simulink model "PMSM_FOC_Tractio"  (R2019b)
settings: Solver=FixedStepAuto  StartTime=0.0  StopTime=10  RelTol=1e-3
model workspace (MAT data in the model file):
  wc : Simulink.Parameter (value not decoded)
values from neighbouring files (symbols this model uses):
  CL_Param = tmp_CL_Param    [PMSM_Parameters.m]
  Cosine_table = [1,0.999995293095708,0.999990587122738,0.999985881149769,0.999981174245477,0.999967055395246,0.999952936545014,0.999938818626106,0.999924698844552,0.999901168979704,0.999877639114857,0.999854108318687,0.999830577522516,0.999797635711730,0.999764694832265,0.999731753021479,0.999698810279369,0.999656459316611,0.999614108353853,0.999571758322418,0.999529405497015,0.999477646313608,0.999425887130201,0 ...(+75635 chars)    [Motor_Table.m]
  ctrlParamsPI = tmp_ctrlParamsPI    [PMSM_Parameters.m]
  Flux_weak = tmp_Fluxweak_struct    [PMSM_Parameters.m]
  Hall_Parameter = tmp_Hall_struct    [PMSM_Parameters.m]
  HFI = tmp_HFI_struct    [PMSM_Parameters.m]
  inverter = struct    [PMSM_Parameters.m]
  MTPA_id_table = [-1.39452500000000,-1.36697494250000,-1.33970177000000,-1.31270548250000,-1.28598608000000,-1.25954356250000,-1.23337793000000,-1.20748918250000,-1.18187732000000,-1.15654234250000,-1.13148425000000,-1.10670304250000,-1.08219872000000,-1.05797128250000,-1.03402073000000,-1.01034706250000,-0.986950280000000,-0.963830382500000,-0.940987370000000,-0.918421242500000,-0.896132000000000,-0.8741196425000 ...(+3439 chars)    [Motor_Table.m]
  MTPA_iq_table = [-10.2740250000000,-10.1791705677750,-10.0840783722000,-9.98875081492500,-9.89319029760000,-9.79739922187500,-9.70137998940000,-9.60513500182500,-9.50866666080000,-9.41197736797500,-9.31506952500000,-9.21794553352500,-9.12060779520000,-9.02305871167500,-8.92530068460000,-8.82733611562500,-8.72916740640000,-8.63079695857500,-8.53222717380000,-8.43346045372500,-8.33449920000000,-8.23534581427500,-8. ...(+3121 chars)    [Motor_Table.m]
  MTPA_Te_Max = single(1.50)    [Motor_Table.m]
  MTPA_Te_Min = single(-1.50)    [Motor_Table.m]
  OPL_Param = tmp_OPL_Param    [PMSM_Parameters.m]
  pmsm = struct    [PMSM_Parameters.m]
  Resolver_Parameter = tmp_Resolver_struct    [PMSM_Parameters.m]
  Sine_table = [0,0.00153398793190718,0.00306797679513693,0.00460196565836668,0.00613595545291901,0.00766988657414913,0.00920381769537926,0.0107377488166094,0.0122716808691621,0.0138054965063930,0.0153393121436238,0.0168731296434999,0.0184069443494082,0.0199405867606401,0.0214742291718721,0.0230078706517816,0.0245415139943361,0.0260749254375696,0.0276083368808031,0.0291417483240366,0.0306751597672701,0.032208281 ...(+75648 chars)    [Motor_Table.m]
  SMO = temp_SMO    [PMSM_Parameters.m]
undefined symbols (not defined in the file or in its folder): DiscIntNeverNeededParam, Kiv, Kiw, Kpv, Kpw, magnitude, sigbuilder_block, SVPWM, Vdc
libraries: powerlib x29, fl_lib x18, simulink x10, nesl_utility x7, eeGeneralControl x4, dspstat3 x3, eeDiscretePi x2, powerlib_extras x1, ee_lib x1
(part 4 of 6)

== system PMSM_FOC_Tractio/Motor_Control/Motor_Control_Funtion/FOC_Control_100us/FOC/D_Current_PI ==
  Current_Command : Inport
  Current_Measured : Inport  Port=2
  Add2 : Sum  Inputs=|+-
  ID_Control : Subsystem
  Vd_voltage : Outport  VectorParamsAs1DForOutWhenUnconnected=off
  wires:
  Current_Command/1 -> Add2/1
  Current_Measured/1 -> Add2/2
  Add2/1 -> ID_Control/1(Err)  "currentControlError"
  ID_Control/1(PI_Out) -> Vd_voltage/1

== system PMSM_FOC_Tractio/Motor_Control/Motor_Control_Funtion/FOC_Control_100us/FOC/Flux_weakening  ==
  Enable : Inport
  Vd : Inport  Port=2
  Vq : Inport  Port=3
  Id : Inport  Port=4
  Iq : Inport  Port=5
  If1 : If  IfExpression=u1 ==1
  Merge : Merge
  Merge1 : Merge
  Subsystem : Subsystem
  Subsystem1 : Subsystem
  Id_ref : Outport
  Iq_ref : Outport  Port=2
  wires:
  Enable/1 -> If1/1
  If1/1 -> Subsystem/Action
  If1/2 -> Subsystem1/Action
  Id/1 -> Subsystem/3(Id), Subsystem1/1(Id)
  Iq/1 -> Subsystem/4(Iq), Subsystem1/2(Iq)
  Vd/1 -> Subsystem/1(Vd)
  Vq/1 -> Subsystem/2(Vq)
  Subsystem/1(Id_ref) -> Merge/1
  Subsystem1/1(Id_ref) -> Merge/2
  Subsystem/2(Iq_ref) -> Merge1/1
  Subsystem1/2(Iq_ref) -> Merge1/2
  Merge1/1 -> Iq_ref/1
  Merge/1 -> Id_ref/1

== system PMSM_FOC_Tractio/Motor_Control/Motor_Control_Funtion/FOC_Control_100us/FOC/HF_Observer ==
  Ialpha-beta : Inport
  Phase_CurrentABC : Inport  Port=2  PortDimensions=3
  Id : Inport  Port=3
  HFI_Enalble : Constant  Value=HFI.Func_Enable  OutDataTypeStr=uint8
  HFI_Function : Subsystem
      settings: RTWSystemCode=Nonreusable function  RTWFcnNameOpts=Use subsystem name
  If1 : If  IfExpression=u1==1  ShowElse=off
  RUN_State : Outport
  HFI_State : Outport  Port=2
  HFI_signal : Outport  Port=3
  speed_est : Outport  Port=4
  theta_est : Outport  Port=5
  Ualpha : Outport  Port=6
  Ubeta : Outport  Port=7
  IPD_Theta : Outport  Port=8
  wires:
  HFI_Function/1(RUN_State) -> RUN_State/1
  HFI_Function/3(HFI_signal) -> HFI_signal/1
  HFI_Function/4(speed_est) -> speed_est/1
  HFI_Function/5(theta_est) -> theta_est/1
  HFI_Function/7(Ubeta) -> Ubeta/1
  HFI_Function/6(Ualpha) -> Ualpha/1
  Id/1 -> HFI_Function/3(Id)
  Phase_CurrentABC/1 -> HFI_Function/2(Phase_CurrentABC)  "Phase_CurrentABC"
  Ialpha-beta/1 -> HFI_Function/1(Ialpha-beta)
  HFI_Enalble/1 -> If1/1
  If1/1 -> HFI_Function/Action
  HFI_Function/2(HFI_State) -> HFI_State/1
  HFI_Function/8(IPD_Theta) -> IPD_Theta/1

== system PMSM_FOC_Tractio/Motor_Control/Motor_Control_Funtion/FOC_Control_100us/FOC/Inverse_Park_Transform ==
  D : Inport
  Q : Inport  Port=2
  Sin_Coefficient : Inport  Port=3
  Cos_Coefficient : Inport  Port=4
  Add1 : Sum  Inputs=+-  OutDataTypeStr=Inherit: Same as first input
  Add2 : Sum  OutDataTypeStr=Inherit: Same as first input
  Cos_Coefficient1 : InportShadow  Port=4
  Product{1..4} (4 alike) : Product  RndMeth=Simplest  OutDataTypeStr=Inherit: Same as first input
  Sin_Coefficient1 : InportShadow  Port=3
  Alpha : Outport  VectorParamsAs1DForOutWhenUnconnected=off
  Beta : Outport  Port=2  VectorParamsAs1DForOutWhenUnconnected=off
  wires:
  Add2/1 -> Beta/1
  Add1/1 -> Alpha/1
  Product3/1 -> Add2/1
  Product4/1 -> Add2/2
  Product1/1 -> Add1/1
  Product2/1 -> Add1/2
  Cos_Coefficient1/1 -> Product4/2
  Sin_Coefficient/1 -> Product2/2
  D/1 -> Product3/1, Product1/1
  Q/1 -> Product2/1, Product4/1
  Sin_Coefficient1/1 -> Product3/2
  Cos_Coefficient/1 -> Product1/2

== system PMSM_FOC_Tractio/Motor_Control/Motor_Control_Funtion/FOC_Control_100us/FOC/Park_Transform ==
  Alpha : Inport
  Beta : Inport  Port=2
  Sin_Coefficient : Inport  Port=3
  Cos_Coefficient : Inport  Port=4
  Add1 : Sum  OutDataTypeStr=Inherit: Same as first input
  Add2 : Sum  Inputs=-+  OutDataTypeStr=Inherit: Same as first input
  Alpha1 : InportShadow
  Beta1 : InportShadow  Port=2
  Cos_Coefficient1 : InportShadow  Port=4
  Produc3t : Product  RndMeth=Simplest  OutDataTypeStr=Inherit: Same as first input
  Product1 : Product  RndMeth=Simplest  OutDataTypeStr=Inherit: Same as first input
  Product2 : Product  RndMeth=Simplest  OutDataTypeStr=Inherit: Same as first input
  Product4 : Product  RndMeth=Simplest  OutDataTypeStr=Inherit: Same as first input
  Sin_Coefficient1 : InportShadow  Port=3
  D : Outport  VectorParamsAs1DForOutWhenUnconnected=off
  Q : Outport  Port=2  VectorParamsAs1DForOutWhenUnconnected=off
  wires:
  Produc3t/1 -> Add2/1
  Product4/1 -> Add2/2
  Product1/1 -> Add1/1
  Product2/1 -> Add1/2
  Alpha1/1 -> Produc3t/1
  Sin_Coefficient1/1 -> Produc3t/2
  Cos_Coefficient1/1 -> Product4/2
  Beta1/1 -> Product4/1
  Alpha/1 -> Product1/1
  Cos_Coefficient/1 -> Product1/2
  Beta/1 -> Product2/1
  Sin_Coefficient/1 -> Product2/2
  Add1/1 -> D/1
  Add2/1 -> Q/1

== system PMSM_FOC_Tractio/Motor_Control/Motor_Control_Funtion/FOC_Control_100us/FOC/Q_Current_PI ==
  Current_Command : Inport
  Current_Measured : Inport  Port=2
  Add2 : Sum  Inputs=|+-
  IQ_Control : Subsystem
  Vq_voltage : Outport  VectorParamsAs1DForOutWhenUnconnected=off
  wires:
  Current_Command/1 -> Add2/1
  Current_Measured/1 -> Add2/2
  Add2/1 -> IQ_Control/1(Err)  "currentControlError"
  IQ_Control/1(PI_Out) -> Vq_voltage/1

== system PMSM_FOC_Tractio/Motor_Control/Motor_Control_Funtion/FOC_Control_100us/FOC/SVPWM ==
  Valpha : Inport
  Vbeta : Inport  Port=2
  Vdc : Inport  Port=3
  Ts : Inport  Port=4
  Gain : Gain  Gain=83990000
  Gain2 : Gain  Gain=83990000
  Gain3 : Gain  Gain=83990000
  N Sector  Caculate : Subsystem  TreatAsAtomicUnit=on
  T1 T2  Caculate : Subsystem  TreatAsAtomicUnit=on
  Tcm calculate : Subsystem  TreatAsAtomicUnit=on
  XYZ Caculate : Subsystem  TreatAsAtomicUnit=on
  Ta : Outport
  Tb : Outport  Port=2
  Tc : Outport  Port=3
  wires:
  Tcm calculate/2(Tcm2) -> Gain2/1
  Tcm calculate/3(Tcm3) -> Gain3/1
  Tcm calculate/1(Tcm1) -> Gain/1
  T1 T2  Caculate/2(T2) -> Tcm calculate/3(T2)
  XYZ Caculate/1(X) -> T1 T2  Caculate/2(X)
  N Sector  Caculate/1(N) -> T1 T2  Caculate/1(N), Tcm calculate/1(N)
  Vdc/1 -> XYZ Caculate/3(Udc)
  T1 T2  Caculate/1(T1) -> Tcm calculate/2(T1)
  XYZ Caculate/3(Z) -> T1 T2  Caculate/4(Z)
  XYZ Caculate/2(Y) -> T1 T2  Caculate/3(Y)
  Valpha/1 -> N Sector  Caculate/2(Ualf), XYZ Caculate/1(Ualfpa)
  Vbeta/1 -> N Sector  Caculate/1(Ubelta), XYZ Caculate/2(Ubelta)
  Ts/1 -> T1 T2  Caculate/5(Tpwm), Tcm calculate/4(Tpwm), XYZ Caculate/4(Tpwm)
  Gain/1 -> Ta/1
  Gain3/1 -> Tc/1
  Gain2/1 -> Tb/1

== system PMSM_FOC_Tractio/Motor_Control/Motor_Control_Funtion/FOC_Control_100us/FOC/Set_Idq ==
  HFI_state : Inport
  Id_Command : Inport  Port=2
  Iq_Command : Inport  Port=3
  Constant1 : Constant  Value=0  OutDataTypeStr=single
  Constant2 : Constant  Value=0  OutDataTypeStr=single
  If1 : If  IfExpression=u1==2 | u1==1
  Merge : Merge
  Merge1 : Merge
  Set_Idq : Subsystem  TreatAsAtomicUnit=on
      settings: RTWSystemCode=Nonreusable function  RTWFcnNameOpts=Use subsystem name
  Set_Idq1 : Subsystem  TreatAsAtomicUnit=on
      settings: RTWSystemCode=Nonreusable function  RTWFcnNameOpts=Use subsystem name
  Id : Outport  VectorParamsAs1DForOutWhenUnconnected=off
  Iq : Outport  Port=2  VectorParamsAs1DForOutWhenUnconnected=off
  wires:
  HFI_state/1 -> If1/1
  Constant2/1 -> Set_Idq/1(Id_Command)
  Constant1/1 -> Set_Idq/2(Iq_Command)
  Id_Command/1 -> Set_Idq1/1(Id_Command)
  Iq_Command/1 -> Set_Idq1/2(Iq_Command)
  If1/1 -> Set_Idq/Action
  If1/2 -> Set_Idq1/Action
  Set_Idq/1(Id) -> Merge/1
  Set_Idq1/1(Id) -> Merge/2
  Merge/1 -> Id/1
  Set_Idq/2(Iq) -> Merge1/1
  Set_Idq1/2(Iq) -> Merge1/2
  Merge1/1 -> Iq/1

== system PMSM_FOC_Tractio/Motor_Control/Motor_Control_Funtion/FOC_Control_100us/FOC/Sine_Cosine ==
  note: Sine Cosine Coefficients
  P : Inport
  Cosine : Lookup_n-D  NumberOfTableDimensions=1  LookupTableObject=''  BreakpointsForDimension1=[0:2*pi/4095:2*pi]  BreakpointsForDimension1FirstPoint=10  BreakpointsForDimension2FirstPoint=10  BreakpointsForDimension1Spacing=12  BreakpointsForDimension2Spacing=12  IndexSearchMethod=Evenly spaced points  Table=Cosine_table  InterpMethod=Flat  DiagnosticForOutOfRangeInput=Error  InternalRulePriority=Speed  RndMeth=Simplest  InputSameDT=on
  Saturation : Saturate  UpperLimit=2*pi-0.0001  LowerLimit=0+0.0001
  Scope : Scope  NumInputPorts=2
  Sine : Lookup_n-D  NumberOfTableDimensions=1  LookupTableObject=''  BreakpointsForDimension1=[0:2*pi/4095:2*pi]  BreakpointsForDimension1FirstPoint=10  BreakpointsForDimension2FirstPoint=10  BreakpointsForDimension1Spacing=12  BreakpointsForDimension2Spacing=12  IndexSearchMethod=Evenly spaced points  Table=Sine_table  InterpMethod=Flat  DiagnosticForOutOfRangeInput=Error  InternalRulePriority=Speed  RndMeth=Simplest  InputSameDT=on
  Sin : Outport  VectorParamsAs1DForOutWhenUnconnected=off
  Cos : Outport  Port=2  VectorParamsAs1DForOutWhenUnconnected=off
  wires:
  P/1 -> Saturation/1  "position"
  Sine/1 -> Scope/1, Sin/1
  Cosine/1 -> Scope/2, Cos/1
  Saturation/1 -> Cosine/1, Sine/1

== system PMSM_FOC_Tractio/Motor_Control/Motor_Control_Funtion/FOC_Control_100us/FOC/Subsystem1 ==
  HFI_State : Inport
  HFI_Ualpha : Inport  Port=2
  HFI_Ubeta : Inport  Port=3
  Ualpha : Inport  Port=4
  Ubeta : Inport  Port=5
  If Action Subsystem1 : Subsystem  TreatAsAtomicUnit=on
  If Action Subsystem2 : Subsystem  TreatAsAtomicUnit=on
  If1 : If  IfExpression=(u1<3)&(u1>0)
  Merge : Merge
  Merge1 : Merge
  Ualpha_out : Outport
  Ubeta_out : Outport  Port=2
  wires:
  If1/1 -> If Action Subsystem2/Action
  If1/2 -> If Action Subsystem1/Action
  HFI_Ualpha/1 -> If Action Subsystem2/1(In1)
  HFI_Ubeta/1 -> If Action Subsystem2/2(In2)
  Ualpha/1 -> If Action Subsystem1/1(In1)
  Ubeta/1 -> If Action Subsystem1/2(In2)
  If Action Subsystem2/1(Out1) -> Merge/1
  If Action Subsystem1/1(Out1) -> Merge/2
  If Action Subsystem2/2(Out2) -> Merge1/1
  If Action Subsystem1/2(Out2) -> Merge1/2
  Merge/1 -> Ualpha_out/1
  Merge1/1 -> Ubeta_out/1
  HFI_State/1 -> If1/1

== system PMSM_FOC_Tractio/Motor_Control/Motor_Control_Funtion/FOC_Control_100us/Iq_selector/Subsystem ==
  In1 : Inport
  Action Port : ActionPort  ActionPortLabel=if(u1 ==2 | u1 ==3)
  Out1 : Outport
  wires:
  In1/1 -> Out1/1

== system PMSM_FOC_Tractio/Motor_Control/Motor_Control_Funtion/FOC_Control_100us/Iq_selector/Subsystem1 ==
  In1 : Inport
  Action Port : ActionPort  ActionPortLabel=else
  Out1 : Outport
  wires:
  In1/1 -> Out1/1

== system PMSM_FOC_Tractio/PMSM/Control/Control/Commutation/Bit concatenate ==
  u : Inport
  Gain : Gain  Gain=[4 2 1]  Multiplication=Matrix(K*u)
  Sum of Elements : Sum  Inputs=+
  y : Outport  VectorParamsAs1DForOutWhenUnconnected=off
  wires:
  u/1 -> Gain/1
  Gain/1 -> Sum of Elements/1
  Sum of Elements/1 -> y/1

== system PMSM_FOC_Tractio/PMSM/SpeedAndAngle/ACC_OMG/Six_point/Sector_1 ==
  Action Port : ActionPort  ActionPortLabel=case [ 1 ]:
  Add : Sum
  Constant : Constant  Value=Hall_Parameter.Sector_1  OutDataTypeStr=single
  Constant1 : Constant  Value=Hall_Parameter.shift  OutDataTypeStr=single
  Angle_0 : Outport
  wires:
  Constant/1 -> Add/1
  Constant1/1 -> Add/2
  Add/1 -> Angle_0/1

== system PMSM_FOC_Tractio/PMSM/SpeedAndAngle/ACC_OMG/Six_point/Sector_2 ==
  Action Port : ActionPort  ActionPortLabel=case [ 2 ]:
  Add : Sum
  Constant1 : Constant  Value=Hall_Parameter.shift  OutDataTypeStr=single
  Pi/3 : Constant  Value=Hall_Parameter.Sector_2  OutDataTypeStr=single
  Angle_0 : Outport
  wires:
  Pi/3/1 -> Add/1
  Constant1/1 -> Add/2
  Add/1 -> Angle_0/1

== system PMSM_FOC_Tractio/PMSM/SpeedAndAngle/ACC_OMG/Six_point/Sector_3 ==
  Action Port : ActionPort  ActionPortLabel=case [ 3 ]:
  Add : Sum
  Constant : Constant  Value=Hall_Parameter.Sector_3  OutDataTypeStr=single
  Constant1 : Constant  Value=Hall_Parameter.shift  OutDataTypeStr=single
  Angle_0 : Outport
  wires:
  Constant/1 -> Add/1
  Add/1 -> Angle_0/1
  Constant1/1 -> Add/2

== system PMSM_FOC_Tractio/PMSM/SpeedAndAngle/ACC_OMG/Six_point/Sector_4 ==
  Action Port : ActionPort  ActionPortLabel=case [ 4 ]:
  Add : Sum
  Constant : Constant  Value=Hall_Parameter.Sector_4  OutDataTypeStr=single
  Constant1 : Constant  Value=Hall_Parameter.shift  OutDataTypeStr=single
  Angle_0 : Outport
  wires:
  Constant/1 -> Add/1
  Add/1 -> Angle_0/1
  Constant1/1 -> Add/2

== system PMSM_FOC_Tractio/PMSM/SpeedAndAngle/ACC_OMG/Six_point/Sector_5 ==
  Action Port : ActionPort  ActionPortLabel=case [ 5 ]:
  Add : Sum
  Constant : Constant  Value=Hall_Parameter.Sector_5  OutDataTypeStr=single
  Constant1 : Constant  Value=Hall_Parameter.shift  OutDataTypeStr=single
  Angle_0 : Outport
  wires:
  Constant/1 -> Add/1
  Add/1 -> Angle_0/1
  Constant1/1 -> Add/2

== system PMSM_FOC_Tractio/PMSM/SpeedAndAngle/ACC_OMG/Six_point/Sector_6 ==
  Action Port : ActionPort  ActionPortLabel=case [ 6 ]:
  Add : Sum
  Constant : Constant  Value=Hall_Parameter.Sector_6  OutDataTypeStr=single
  Constant1 : Constant  Value=Hall_Parameter.shift  OutDataTypeStr=single
  Angle_0 : Outport
  wires:
  Constant/1 -> Add/1
  Add/1 -> Angle_0/1
  Constant1/1 -> Add/2

== system PMSM_FOC_Tractio/PMSM/SpeedAndAngle/ADC_IRQ/HallAngle_calibration/If Action Subsystem1 ==
  In1 : Inport
  Action Port : ActionPort  ActionPortLabel=else
  Out1 : Outport
  wires:
  In1/1 -> Out1/1

== system PMSM_FOC_Tractio/PMSM/SpeedAndAngle/ADC_IRQ/HallAngle_calibration/If Action Subsystem2 ==
  In1 : Inport
  Action Port : ActionPort  ActionPortLabel=if(u1 > 6.283185307)
  2pi : Constant  Value=2*pi  OutDataTypeStr=single
  Subtract1 : Sum  Inputs=+-  OutDataTypeStr=single
  Out1 : Outport
  wires:
  In1/1 -> Subtract1/1
  Subtract1/1 -> Out1/1
  2pi/1 -> Subtract1/2

== system PMSM_FOC_Tractio/PMSM/SpeedAndAngle/ADC_IRQ/HallAngle_calibration/If Action Subsystem3 ==
  In1 : Inport
  Action Port : ActionPort  ActionPortLabel=elseif(u1<0)
  Angle_offset : Constant  Value=2*pi  OutDataTypeStr=single
  Subtract1 : Sum
  Out1 : Outport
  wires:
  In1/1 -> Subtract1/1
  Subtract1/1 -> Out1/1
  Angle_offset/1 -> Subtract1/2

== system PMSM_FOC_Tractio/Motor_Control/Motor_Control_Funtion/Angle_Speed_100us/Resolver_Observer/Angle_calibration/If Action Subsystem1 ==
  In1 : Inport
  Action Port : ActionPort  ActionPortLabel=else
  Out1 : Outport
  wires:
  In1/1 -> Out1/1

== system PMSM_FOC_Tractio/Motor_Control/Motor_Control_Funtion/Angle_Speed_100us/Resolver_Observer/Angle_calibration/If Action Subsystem2 ==
  In1 : Inport
  Action Port : ActionPort  ActionPortLabel=if(u1 > 6.283185307)
  2pi : Constant  Value=2*pi  OutDataTypeStr=single
  Subtract1 : Sum  Inputs=+-  OutDataTypeStr=single
  Out1 : Outport
  wires:
  In1/1 -> Subtract1/1
  Subtract1/1 -> Out1/1
  2pi/1 -> Subtract1/2

== system PMSM_FOC_Tractio/Motor_Control/Motor_Control_Funtion/Angle_Speed_100us/Resolver_Observer/Angle_calibration/If Action Subsystem3 ==
  In1 : Inport
  Action Port : ActionPort  ActionPortLabel=elseif(u1<0)
  Angle_offset : Constant  Value=2*pi  OutDataTypeStr=single
  Subtract1 : Sum
  Out1 : Outport
  wires:
  In1/1 -> Subtract1/1
  Subtract1/1 -> Out1/1
  Angle_offset/1 -> Subtract1/2

== system PMSM_FOC_Tractio/Motor_Control/Motor_Control_Funtion/Angle_Speed_100us/Resolver_Observer/Resolver_Angle_cacl/Sine_Cosine ==
  note: Sine Cosine Coefficients
  P : Inport
  Cosine : Lookup_n-D  NumberOfTableDimensions=1  LookupTableObject=''  BreakpointsForDimension1=[0:2*pi/4095:2*pi]  BreakpointsForDimension1FirstPoint=10  BreakpointsForDimension2FirstPoint=10  BreakpointsForDimension1Spacing=12  BreakpointsForDimension2Spacing=12  IndexSearchMethod=Evenly spaced points  Table=Cosine_table  InterpMethod=Flat  DiagnosticForOutOfRangeInput=Error  InternalRulePriority=Speed  RndMeth=Simplest  InputSameDT=on
  Saturation : Saturate  UpperLimit=2*pi-0.0001  LowerLimit=0+0.0001
  Scope : Scope  NumInputPorts=2
  Sine : Lookup_n-D  NumberOfTableDimensions=1  LookupTableObject=''  BreakpointsForDimension1=[0:2*pi/4095:2*pi]  BreakpointsForDimension1FirstPoint=10  BreakpointsForDimension2FirstPoint=10  BreakpointsForDimension1Spacing=12  BreakpointsForDimension2Spacing=12  IndexSearchMethod=Evenly spaced points  Table=Sine_table  InterpMethod=Flat  DiagnosticForOutOfRangeInput=Error  InternalRulePriority=Speed  RndMeth=Simplest  InputSameDT=on
  Sin : Outport  VectorParamsAs1DForOutWhenUnconnected=off
  Cos : Outport  Port=2  VectorParamsAs1DForOutWhenUnconnected=off
  wires:
  P/1 -> Saturation/1  "position"
  Sine/1 -> Scope/1, Sin/1
  Cosine/1 -> Scope/2, Cos/1
  Saturation/1 -> Cosine/1, Sine/1

== system PMSM_FOC_Tractio/Motor_Control/Motor_Control_Funtion/Angle_Speed_100us/SMO/Angle_calibration/If Action Subsystem1 ==
  In1 : Inport
  Action Port : ActionPort  ActionPortLabel=else
  Out1 : Outport
  wires:
  In1/1 -> Out1/1

== system PMSM_FOC_Tractio/Motor_Control/Motor_Control_Funtion/Angle_Speed_100us/SMO/Angle_calibration/If Action Subsystem2 ==
  In1 : Inport
  Action Port : ActionPort  ActionPortLabel=if(u1 > 6.283185307)
  2pi : Constant  Value=2*pi  OutDataTypeStr=single
  Subtract1 : Sum  Inputs=+-  OutDataTypeStr=single
  Out1 : Outport
  wires:
  In1/1 -> Subtract1/1
  Subtract1/1 -> Out1/1
  2pi/1 -> Subtract1/2

== system PMSM_FOC_Tractio/Motor_Control/Motor_Control_Funtion/Angle_Speed_100us/SMO/Angle_calibration/If Action Subsystem3 ==
  In1 : Inport
  Action Port : ActionPort  ActionPortLabel=elseif(u1<0)
  Angle_offset : Constant  Value=2*pi  OutDataTypeStr=single
  Subtract1 : Sum
  Out1 : Outport
  wires:
  In1/1 -> Subtract1/1
  Subtract1/1 -> Out1/1
  Angle_offset/1 -> Subtract1/2

== system PMSM_FOC_Tractio/Motor_Control/Motor_Control_Funtion/Angle_Speed_100us/SMO/Delta_theta/Sine_Cosine ==
  note: Sine Cosine Coefficients
  P : Inport
  Cosine : Lookup_n-D  NumberOfTableDimensions=1  LookupTableObject=''  BreakpointsForDimension1=[0:2*pi/4095:2*pi]  BreakpointsForDimension1FirstPoint=10  BreakpointsForDimension2FirstPoint=10  BreakpointsForDimension1Spacing=12  BreakpointsForDimension2Spacing=12  IndexSearchMethod=Evenly spaced points  Table=Cosine_table  InterpMethod=Flat  DiagnosticForOutOfRangeInput=Error  InternalRulePriority=Speed  RndMeth=Simplest  InputSameDT=on
  Saturation : Saturate  UpperLimit=2*pi-0.0001  LowerLimit=0+0.0001
  Scope : Scope  NumInputPorts=2
  Sine : Lookup_n-D  NumberOfTableDimensions=1  LookupTableObject=''  BreakpointsForDimension1=[0:2*pi/4095:2*pi]  BreakpointsForDimension1FirstPoint=10  BreakpointsForDimension2FirstPoint=10  BreakpointsForDimension1Spacing=12  BreakpointsForDimension2Spacing=12  IndexSearchMethod=Evenly spaced points  Table=Sine_table  InterpMethod=Flat  DiagnosticForOutOfRangeInput=Error  InternalRulePriority=Speed  RndMeth=Simplest  InputSameDT=on
  Sin : Outport  VectorParamsAs1DForOutWhenUnconnected=off
  Cos : Outport  Port=2  VectorParamsAs1DForOutWhenUnconnected=off
  wires:
  P/1 -> Saturation/1  "position"
  Sine/1 -> Scope/1, Sin/1
  Cosine/1 -> Scope/2, Cos/1
  Saturation/1 -> Cosine/1, Sine/1

== system PMSM_FOC_Tractio/Motor_Control/Motor_Control_Funtion/Angle_Speed_100us/SMO/Ealphabeta_Ca1/If Action Subsystem1 ==
  In1 : Inport
  Action Port : ActionPort  ActionPortLabel=if(u1>u2)
  Zalpha : Outport  VectorParamsAs1DForOutWhenUnconnected=off
  wires:
  In1/1 -> Zalpha/1

== system PMSM_FOC_Tractio/Motor_Control/Motor_Control_Funtion/Angle_Speed_100us/SMO/Ealphabeta_Ca1/If Action Subsystem2 ==
  In1 : Inport
  Action Port : ActionPort  ActionPortLabel=elseif(u1<u3)
  Zalpha : Outport  VectorParamsAs1DForOutWhenUnconnected=off
  wires:
  In1/1 -> Zalpha/1

== system PMSM_FOC_Tractio/Motor_Control/Motor_Control_Funtion/Angle_Speed_100us/SMO/Ealphabeta_Ca1/If Action Subsystem3 ==
  In1 : Inport
  Action Port : ActionPort  ActionPortLabel=else
  Constant : Constant  Value=SMO.tao  OutDataTypeStr=single
  Divide : Product  Inputs=*/
  Zalpha : Outport  VectorParamsAs1DForOutWhenUnconnected=off
  wires:
  In1/1 -> Divide/1
  Divide/1 -> Zalpha/1
  Constant/1 -> Divide/2

== system PMSM_FOC_Tractio/Motor_Control/Motor_Control_Funtion/Angle_Speed_100us/SMO/Ealphabeta_Ca1/If Action Subsystem4 ==
  In1 : Inport
  Action Port : ActionPort  ActionPortLabel=if(u1>u2)
  Zbeta : Outport  VectorParamsAs1DForOutWhenUnconnected=off
  wires:
  In1/1 -> Zbeta/1

== system PMSM_FOC_Tractio/Motor_Control/Motor_Control_Funtion/Angle_Speed_100us/SMO/Ealphabeta_Ca1/If Action Subsystem5 ==
  In1 : Inport
  Action Port : ActionPort  ActionPortLabel=elseif(u1<u3)
  Zbeta : Outport  VectorParamsAs1DForOutWhenUnconnected=off
  wires:
  In1/1 -> Zbeta/1

== system PMSM_FOC_Tractio/Motor_Control/Motor_Control_Funtion/Angle_Speed_100us/SMO/Ealphabeta_Ca1/If Action Subsystem6 ==
  In1 : Inport
  Action Port : ActionPort  ActionPortLabel=else
  Constant : Constant  Value=SMO.tao
  Divide : Product  Inputs=*/
  Zbeta : Outport  VectorParamsAs1DForOutWhenUnconnected=off
  wires:
  In1/1 -> Divide/1
  Divide/1 -> Zbeta/1
  Constant/1 -> Divide/2

== system PMSM_FOC_Tractio/Motor_Control/Motor_Control_Funtion/Angle_Speed_100us/SpeedAndAngle/ACC_OMG/BLDC ==
  Hall : Inport
  We : Inport  Port=2
  BLDC_State : Inport  Port=3
  Control : Subsystem
  Low pass filter : DiscreteTransferFcn  Numerator=[1-exp(-2*pi*20*inverter.Ts)]  Denominator=[1 -exp(-2*pi*20*inverter.Ts)]
  Scope : Scope  NumInputPorts=2
  T3 : Constant  Value=1000
  Gate : Outport  VectorParamsAs1DForOutWhenUnconnected=off
  Duty : Outport  Port=2  VectorParamsAs1DForOutWhenUnconnected=off
  wires:
  Hall/1 -> Control/3(Hall)
  T3/1 -> Control/1(RPMReq)
  We/1 -> Scope/2, Low pass filter/1
  Control/1(Gate) -> Gate/1
  Control/2(Duty) -> Duty/1
  Low pass filter/1 -> Scope/1, Control/2(w_sens)
  BLDC_State/1 -> Control/4(BLDC_State)

== system PMSM_FOC_Tractio/Motor_Control/Motor_Control_Funtion/Angle_Speed_100us/SpeedAndAngle/ACC_OMG/Six_point ==
  In1 : Inport
  Merge2 : Merge  Inputs=6
  Scope : Scope  NumInputPorts=2
  Sector_1 : Subsystem
  Sector_2 : Subsystem
  Sector_3 : Subsystem
  Sector_4 : Subsystem
  Sector_5 : Subsystem
  Sector_6 : Subsystem
  Switch Case2 : SwitchCase  CaseConditions={1,2,3,4,5,6}  ShowDefaultCase=off
  Out1 : Outport
  wires:
  Sector_4/1(Angle_0) -> Merge2/4
  Switch Case2/5 -> Sector_5/Action
  Sector_6/1(Angle_0) -> Merge2/6
  Sector_5/1(Angle_0) -> Merge2/5
  Switch Case2/6 -> Sector_6/Action
  Switch Case2/3 -> Sector_3/Action
  Switch Case2/4 -> Sector_4/Action
  Sector_1/1(Angle_0) -> Merge2/1
  Switch Case2/2 -> Sector_2/Action
  In1/1 -> Scope/1, Switch Case2/1
  Sector_3/1(Angle_0) -> Merge2/3
  Switch Case2/1 -> Sector_1/Action
  Sector_2/1(Angle_0) -> Merge2/2
  Merge2/1 -> Scope/2, Out1/1

== system PMSM_FOC_Tractio/Motor_Control/Motor_Control_Funtion/Angle_Speed_100us/SpeedAndAngle/ADC_IRQ/HallAngle_calibration ==
  Angle_input : Inport
  Angle_offset : Constant  Value=Hall_Parameter.shift
  If Action Subsystem1 : Subsystem  TreatAsAtomicUnit=on
  If Action Subsystem2 : Subsystem  TreatAsAtomicUnit=on
  If Action Subsystem3 : Subsystem  TreatAsAtomicUnit=on
  If1 : If  IfExpression=u1 > 6.283185307  ElseIfExpressions=u1<0
  Merge1 : Merge  Inputs=3
  Subtract1 : Sum
  Angle_output : Outport
  wires:
  Angle_input/1 -> Subtract1/1
  Angle_offset/1 -> Subtract1/2  "Control_ModeCommand"
  If1/1 -> If Action Subsystem2/Action
  If1/3 -> If Action Subsystem1/Action
  If Action Subsystem2/1(Out1) -> Merge1/1
  Subtract1/1 -> If Action Subsystem3/1(In1), If Action Subsystem1/1(In1), If Action Subsystem2/1(In1), If1/1
  If Action Subsystem1/1(Out1) -> Merge1/3
  If Action Subsystem3/1(Out1) -> Merge1/2
  If1/2 -> If Action Subsystem3/Action
  Merge1/1 -> Angle_output/1

== system PMSM_FOC_Tractio/Motor_Control/Motor_Control_Funtion/Angle_Speed_100us/SpeedAndAngle/Subsystem/Subsystem ==
  Action Port : ActionPort  ActionPortLabel=if(u1 ==1)
  Commutation : Subsystem
  Duty : Constant  Value=0.7*4200  SampleTime=-1
  Gate : Outport  VectorParamsAs1DForOutWhenUnconnected=off
  Duty_Set : Outport  Port=2  VectorParamsAs1DForOutWhenUnconnected=off
  wires:
  Duty/1 -> Duty_Set/1
  Commutation/1(S) -> Gate/1

== system PMSM_FOC_Tractio/Motor_Control/Motor_Control_Funtion/Angle_Speed_100us/SpeedAndAngle/Subsystem/Subsystem1 ==
  Hall : Inport
  Action Port : ActionPort  ActionPortLabel=elseif(u1 ==2)
  Commutation : Subsystem
  Duty : Constant  Value=0.7*4200  SampleTime=-1
  Gate : Outport  VectorParamsAs1DForOutWhenUnconnected=off
  Duty_Set : Outport  Port=2  VectorParamsAs1DForOutWhenUnconnected=off
  wires:
  Duty/1 -> Duty_Set/1
  Hall/1 -> Commutation/1(Hall)
  Commutation/1(S) -> Gate/1

== system PMSM_FOC_Tractio/Motor_Control/Motor_Control_Funtion/Angle_Speed_100us/SpeedAndAngle/Subsystem1/Subsystem ==
  In1 : Inport
  In2 : Inport  Port=2
  Action Port : ActionPort  ActionPortLabel=if(u1 ==1 | u1 ==2)
  Out1 : Outport
  Out2 : Outport  Port=2
  wires:
  In1/1 -> Out1/1
  In2/1 -> Out2/1

== system PMSM_FOC_Tractio/Motor_Control/Motor_Control_Funtion/Angle_Speed_100us/SpeedAndAngle/Subsystem1/Subsystem1 ==
  In1 : Inport
  In2 : Inport  Port=2
  Action Port : ActionPort  ActionPortLabel=elseif(u1==3)
  Out1 : Outport
  Out2 : Outport  Port=2
  wires:
  In1/1 -> Out1/1
  In2/1 -> Out2/1

== system PMSM_FOC_Tractio/Motor_Control/Motor_Control_Funtion/Control_Command_2ms/Speed_PI/Speed_PI/Speed_Control ==
  Err : Inport
  Action Port : ActionPort  ActionPortLabel=if((u1==3)&(u2==1))
  Add : Sum
  Cons : Constant  Value=0  OutDataTypeStr=single
  Discrete-Time Integrator : DiscreteIntegrator  SampleTime=-1  ICPrevOutput=DiscIntNeverNeededParam  ICPrevScaledInput=DiscIntNeverNeededParam
  Ki : Constant  Value=ctrlParamsPI.speed_PI_Ki  OutDataTypeStr=single
  Kp : Constant  Value=ctrlParamsPI.speed_PI_Kp  OutDataTypeStr=single
  Product : Product
  Product1 : Product
  Relational Operator1 : RelationalOperator  Operator===  OutDataTypeStr=boolean  RndMeth=Simplest
  Saturation : Saturate  UpperLimit=ctrlParamsPI.speed_PI_OutputMax  LowerLimit=ctrlParamsPI.speed_PI_OutputMin
  Scope : Scope
  Switch : Switch  Criteria=u2 > Threshold
  Unit Delay3 : UnitDelay  SampleTime=-1  HasFrameUpgradeWarning=on
  PI_Out : Outport
  wires:
  Kp/1 -> Product/1
  Err/1 -> Switch/1, Product/2
  Switch/1 -> Product1/2
  Product1/1 -> Discrete-Time Integrator/1
  Product/1 -> Add/1
  Add/1 -> Relational Operator1/1, Saturation/1
  Saturation/1 -> Relational Operator1/2, PI_Out/1
  Discrete-Time Integrator/1 -> Add/2, Scope/1
  Relational Operator1/1 -> Unit Delay3/1
  Ki/1 -> Product1/1
  Unit Delay3/1 -> Switch/2
  Cons/1 -> Switch/3

== system PMSM_FOC_Tractio/Motor_Control/Motor_Control_Funtion/Control_Command_2ms/Speed_PI/Speed_PI/Speed_Control1 ==
  Err : Inport
  Action Port : ActionPort  ActionPortLabel=elseif((u2==0) & ((u3~=2)&(u3~=3)))
  Add : Sum
  Cons : Constant  Value=0  OutDataTypeStr=single
  Discrete-Time Integrator : DiscreteIntegrator  SampleTime=-1  ICPrevOutput=DiscIntNeverNeededParam  ICPrevScaledInput=DiscIntNeverNeededParam
  Ki : Constant  Value=ctrlParamsPI.speed_PI_Ki  OutDataTypeStr=single
  Kp : Constant  Value=ctrlParamsPI.speed_PI_Kp  OutDataTypeStr=single
  Product : Product
  Product1 : Product
  Relational Operator1 : RelationalOperator  Operator===  OutDataTypeStr=boolean  RndMeth=Simplest
  Saturation : Saturate  UpperLimit=ctrlParamsPI.speed_PI_OutputMax  LowerLimit=ctrlParamsPI.speed_PI_OutputMin
  Switch : Switch  Criteria=u2 > Threshold
  Unit Delay3 : UnitDelay  SampleTime=-1  HasFrameUpgradeWarning=on
  PI_Out : Outport
  wires:
  Kp/1 -> Product/1
  Err/1 -> Switch/1, Product/2
  Switch/1 -> Product1/2
  Product1/1 -> Discrete-Time Integrator/1
  Product/1 -> Add/1
  Add/1 -> Relational Operator1/1, Saturation/1
  Saturation/1 -> Relational Operator1/2, PI_Out/1
  Discrete-Time Integrator/1 -> Add/2
  Relational Operator1/1 -> Unit Delay3/1
  Ki/1 -> Product1/1
  Unit Delay3/1 -> Switch/2
  Cons/1 -> Switch/3

== system PMSM_FOC_Tractio/Motor_Control/Motor_Control_Funtion/FOC_Control_100us/FOC/Angle_set/Subsystem ==
  HFI_state : Inport
  HFI_angle : Inport  Port=2
  IPD_Angle : Inport  Port=3
  Action Port : ActionPort  ActionPortLabel=if(u1 ==1)
  If1 : If  IfExpression=u1 ==3  ElseIfExpressions=u1 <3  ShowElse=off
  Merge : Merge
  Subsystem1 : Subsystem
  Subsystem2 : Subsystem
  Out1 : Outport
  wires:
  HFI_state/1 -> If1/1
  HFI_angle/1 -> Subsystem1/1(HFI_Angle)
  If1/2 -> Subsystem2/Action
  If1/1 -> Subsystem1/Action
  IPD_Angle/1 -> Subsystem2/1(IPD_Angle)
  Merge/1 -> Out1/1
  Subsystem1/1(Out1) -> Merge/1
  Subsystem2/1(Out1) -> Merge/2

== system PMSM_FOC_Tractio/Motor_Control/Motor_Control_Funtion/FOC_Control_100us/FOC/Angle_set/Subsystem1 ==
  Reso_angle : Inport
  Action Port : ActionPort  ActionPortLabel=else
  Out1 : Outport
  wires:
  Reso_angle/1 -> Out1/1

== system PMSM_FOC_Tractio/Motor_Control/Motor_Control_Funtion/FOC_Control_100us/FOC/Clarke_Transform/Clark1 ==
  Iabc : Inport
  Add : Sum  Inputs=+--
  Add1 : Sum  Inputs=+-
  Demux : Demux  Outputs=3
  Gain : Gain  Gain=0.5
  Gain1 : Gain  Gain=0.5
  Gain2 : Gain  Gain=sqrt(2/3)
  Gain3 : Gain  Gain=sqrt(3)/2
  Gain4 : Gain  Gain=sqrt(3)/2
  Gain5 : Gain  Gain=sqrt(2/3)
  Ialpha : Outport  VectorParamsAs1DForOutWhenUnconnected=off
  Ibeta : Outport  Port=2  VectorParamsAs1DForOutWhenUnconnected=off
  wires:
  Iabc/1 -> Demux/1
  Demux/1 -> Add/1
  Gain/1 -> Add/2
  Demux/2 -> Gain3/1, Gain/1
  Gain1/1 -> Add/3
  Demux/3 -> Gain4/1, Gain1/1
  Add/1 -> Gain2/1
  Gain2/1 -> Ialpha/1
  Gain3/1 -> Add1/1
  Gain4/1 -> Add1/2
  Add1/1 -> Gain5/1
  Gain5/1 -> Ibeta/1

== system PMSM_FOC_Tractio/Motor_Control/Motor_Control_Funtion/FOC_Control_100us/FOC/D_Current_PI/ID_Control ==
  Err : Inport
  Add : Sum
  Cons : Constant  Value=0  OutDataTypeStr=single
  Discrete-Time Integrator : DiscreteIntegrator  SampleTime=-1  ICPrevOutput=DiscIntNeverNeededParam  ICPrevScaledInput=DiscIntNeverNeededParam
  Ki : Constant  Value=ctrlParamsPI.ID_Current_PI_Ki  OutDataTypeStr=single
  Kp : Constant  Value=ctrlParamsPI.ID_Current_PI_Kp  OutDataTypeStr=single
  Product : Product
  Product1 : Product
  Relational Operator1 : RelationalOperator  Operator===  OutDataTypeStr=boolean  RndMeth=Simplest
  Saturation : Saturate  UpperLimit=ctrlParamsPI.ID_Current_PI_OutputMax  LowerLimit=ctrlParamsPI.ID_Current_PI_OutputMin
  Switch : Switch  Criteria=u2 > Threshold
  Unit Delay3 : UnitDelay  SampleTime=-1  HasFrameUpgradeWarning=on
  PI_Out : Outport
  wires:
  Kp/1 -> Product/1
  Err/1 -> Switch/1, Product/2
  Switch/1 -> Product1/2
  Product1/1 -> Discrete-Time Integrator/1
  Product/1 -> Add/1
  Add/1 -> Relational Operator1/1, Saturation/1
  Saturation/1 -> Relational Operator1/2, PI_Out/1
  Cons/1 -> Switch/3
  Discrete-Time Integrator/1 -> Add/2
  Relational Operator1/1 -> Unit Delay3/1
  Ki/1 -> Product1/1
  Unit Delay3/1 -> Switch/2

== system PMSM_FOC_Tractio/Motor_Control/Motor_Control_Funtion/FOC_Control_100us/FOC/Flux_weakening /Subsystem ==
  Vd : Inport
  Vq : Inport  Port=2
  Id : Inport  Port=3
  Iq : Inport  Port=4
  Action Port : ActionPort  ActionPortLabel=if(u1 ==1)
  Flux_weak : Subsystem  TreatAsAtomicUnit=on  mask{kp=Flux_weak.Kp, ki=Flux_weak.Ki, Id_max=Flux_weak.Idref_max, Id_min=Flux_weak.Idref_min}
      settings: RTWSystemCode=Nonreusable function  RTWFcnNameOpts=Use subsystem name
  Id_ref : Outport
  Iq_ref : Outport  Port=2
  wires:
  Vd/1 -> Flux_weak/1(Vd)
  Vq/1 -> Flux_weak/2(Vq)
  Id/1 -> Flux_weak/3(id_input)
  Iq/1 -> Flux_weak/4(Iq_input)
  Flux_weak/1(Id_ref) -> Id_ref/1
  Flux_weak/2(iq_ref) -> Iq_ref/1

== system PMSM_FOC_Tractio/Motor_Control/Motor_Control_Funtion/FOC_Control_100us/FOC/Flux_weakening /Subsystem1 ==
  Id : Inport
  Iq : Inport  Port=2
  Action Port : ActionPort  ActionPortLabel=else
  Id_ref : Outport
  Iq_ref : Outport  Port=2
  wires:
  Id/1 -> Id_ref/1
  Iq/1 -> Iq_ref/1

== system PMSM_FOC_Tractio/Motor_Control/Motor_Control_Funtion/FOC_Control_100us/FOC/HF_Observer/HFI_Function ==
  Ialpha-beta : Inport
  Phase_CurrentABC : Inport  Port=2  PortDimensions=3
  Id : Inport  Port=3
  Action Port : ActionPort  ActionPortLabel=if(u1==1)
  Delay : Delay  DelayLength=1  InitialCondition=0
  Delay1 : Delay  DelayLength=1  InitialCondition=0
  Delay2 : Delay  DelayLength=1  InitialCondition=0
  HFI : Subsystem
  HFI_Enalble : Constant  Value=HFI.Func_Enable  OutDataTypeStr=uint8
  HFI_State_machine : Stateflow chart  BlockKeywords=__PRM__SERIALIZED__DATA__:Stateflow Chart,Stateflow Diagram  TreatAsAtomicUnit=on
      settings: RTWSystemCode=Nonreusable function  RTWFcnNameOpts=Use subsystem name
  IPD : Subsystem  TreatAsAtomicUnit=on
      settings: RTWSystemCode=Nonreusable function
  Merge : Merge
  Merge1 : Merge
  Merge2 : Merge
  NS : Subsystem  TreatAsAtomicUnit=on
      settings: RTWSystemCode=Nonreusable function
  Switch Case1 : SwitchCase  CaseConditions={1,2,3}
  RUN_State : Outport
  HFI_State : Outport  Port=2
  HFI_signal : Outport  Port=3
  speed_est : Outport  Port=4
  theta_est : Outport  Port=5
  Ualpha : Outport  Port=6
  Ubeta : Outport  Port=7
  IPD_Theta : Outport  Port=8
  wires:
  NS/1(Ualpha) -> Merge/2
  HFI_State_machine/1(HFI_state) -> HFI_State/1, Switch Case1/1
  Delay/1 -> NS/1(Id)
  Switch Case1/2 -> [NS]
  Id/1 -> Delay/1
  IPD/2(Ubeta) -> Merge1/1
  [NS] -> NS/Action
  HFI/5(theta_est) -> Merge2/2
  IPD/3(Theta) -> Delay1/1
  Phase_CurrentABC/1 -> IPD/1(Iabc)  "Phase_CurrentABC"
  Delay1/1 -> NS/2(Theta)
  HFI/2(speed_est) -> speed_est/1
  Ialpha-beta/1 -> HFI/1(Ialpha-beta)
  Merge1/1 -> Ubeta/1
  Switch Case1/4 -> [default]
  [IPD] -> IPD/Action
  Merge/1 -> Ualpha/1
  [RUN] -> HFI/Action
  NS/2(Ubeta) -> Merge1/2
  Switch Case1/1 -> [IPD]
  HFI_Enalble/1 -> HFI_State_machine/1(HFI_flag)
  HFI/1(HFI_signal) -> HFI_signal/1
  IPD/1(Ualpha) -> Merge/1
  NS/3(IPD_Angle) -> Merge2/1
  Merge2/1 -> theta_est/1
  Switch Case1/3 -> [RUN]
  NS/4(Angle_RUN) -> Delay2/1
  Delay2/1 -> HFI/2(IPD_angle)
  HFI/3(HFI_State) -> RUN_State/1
  HFI/4(IPD_Theta) -> IPD_Theta/1

== system PMSM_FOC_Tractio/Motor_Control/Motor_Control_Funtion/FOC_Control_100us/FOC/Q_Current_PI/IQ_Control ==
  Err : Inport
  Add : Sum
  Cons : Constant  Value=0  OutDataTypeStr=single
  Discrete-Time Integrator : DiscreteIntegrator  SampleTime=-1  ICPrevOutput=DiscIntNeverNeededParam  ICPrevScaledInput=DiscIntNeverNeededParam
  Ki : Constant  Value=ctrlParamsPI.IQ_Current_PI_Ki  OutDataTypeStr=single
  Kp : Constant  Value=ctrlParamsPI.IQ_Current_PI_Kp  OutDataTypeStr=single
  Product : Product
  Product1 : Product
  Relational Operator1 : RelationalOperator  Operator===  OutDataTypeStr=boolean  RndMeth=Simplest
  Saturation : Saturate  UpperLimit=ctrlParamsPI.IQ_Current_PI_OutputMax  LowerLimit=ctrlParamsPI.IQ_Current_PI_OutputMin
  Switch : Switch  Criteria=u2 > Threshold
  Unit Delay3 : UnitDelay  SampleTime=-1  HasFrameUpgradeWarning=on
  PI_Out : Outport
  wires:
  Kp/1 -> Product/1
  Err/1 -> Switch/1, Product/2
  Switch/1 -> Product1/2
  Product1/1 -> Discrete-Time Integrator/1
  Product/1 -> Add/1
  Add/1 -> Relational Operator1/1, Saturation/1
  Saturation/1 -> Relational Operator1/2, PI_Out/1
  Cons/1 -> Switch/3
  Discrete-Time Integrator/1 -> Add/2
  Relational Operator1/1 -> Unit Delay3/1
  Ki/1 -> Product1/1
  Unit Delay3/1 -> Switch/2

== system PMSM_FOC_Tractio/Motor_Control/Motor_Control_Funtion/FOC_Control_100us/FOC/SVPWM/N Sector  Caculate ==
  Ubelta : Inport
  Ualf : Inport  Port=2
  Add : Sum  Inputs=+++
  Add1 : Sum  Inputs=-+
  Add2 : Sum  Inputs=--
  Constant : Constant  OutDataTypeStr=single
  Constant1 : Constant  Value=0  OutDataTypeStr=single
  Gain : Gain  Gain=sqrt(3)
  Gain1 : Gain  Gain=2
  Gain2 : Gain  Gain=4
  Saturation : Saturate  UpperLimit=6  LowerLimit=1
  Switch : Switch
  Switch1 : Switch
  Switch2 : Switch
  N : Outport
  wires:
  Saturation/1 -> N/1
  Add/1 -> Saturation/1
  Gain2/1 -> Add/3
  Switch2/1 -> Gain2/1
  Add2/1 -> Switch2/2
  Gain1/1 -> Add/2
  Switch1/1 -> Gain1/1
  Add1/1 -> Switch1/2
  Gain/1 -> Add2/2, Add1/2
  Ualf/1 -> Gain/1
  Switch/1 -> Add/1
  Constant1/1 -> Switch/3, Switch1/3, Switch2/3
  Constant/1 -> Switch/1, Switch1/1, Switch2/1
  Ubelta/1 -> Add2/1, Add1/1, Switch/2

== system PMSM_FOC_Tractio/Motor_Control/Motor_Control_Funtion/FOC_Control_100us/FOC/SVPWM/T1 T2  Caculate ==
  note: Z
  note: Y
  note: -X
  note: X
  note: -Y
  note: Y
  note: -X
  note: X
  note: Z
  note: -Y
  note: -Z
  note: X
  note: Y
  note: Z
  N : Inport
  X : Inport  Port=2
  Y : Inport  Port=3
  Z : Inport  Port=4
  Tpwm : Inport  Port=5
  Add : Sum
  Add1 : Sum  Inputs=-+
  Divide : Product  Inputs=**/
  Divide1 : Product  Inputs=/**
  Gain : Gain  Gain=-1
  Gain1 : Gain  Gain=-1
  Gain2 : Gain  Gain=-1
  Index Vector : MultiPortSwitch  Inputs=6
  Index Vector1 : MultiPortSwitch  Inputs=6
  Switch : Switch  Criteria=u2 > Threshold
  Switch2 : Switch  Criteria=u2 > Threshold
  T1 : Outport
  T2 : Outport  Port=2
  wires:
  Switch2/1 -> T2/1
  Divide1/1 -> Switch2/3
  Switch/1 -> T1/1
  Add1/1 -> Switch/2, Switch2/2
  Add/1 -> Divide1/1, Divide/3, Add1/1
  Tpwm/1 -> Divide1/2, Divide/2, Add1/2
  Divide/1 -> Switch/3
  Index Vector1/1 -> Switch2/1, Add/2, Divide1/3
  Index Vector/1 -> Switch/1, Divide/1, Add/1
  Gain1/1 -> Index Vector/7, Index Vector1/6
  Gain2/1 -> Index Vector/4, Index Vector1/7  "-Z"
  Gain/1 -> Index Vector/5, Index Vector1/3
  Y/1 -> Gain1/1, Index Vector/3, Index Vector1/2
  X/1 -> Index Vector1/4, Index Vector/6, Gain/1
  Z/1 -> Index Vector/2, Index Vector1/5, Gain2/1
  N/1 -> Index Vector1/1, Index Vector/1

== system PMSM_FOC_Tractio/Motor_Control/Motor_Control_Funtion/FOC_Control_100us/FOC/SVPWM/Tcm calculate ==
  note: Tc
  note: Tb
  note: Ta
  N : Inport
  T1 : Inport  Port=2
  T2 : Inport  Port=3
  Tpwm : Inport  Port=4
  Add : Sum  Inputs=--+
  Add1 : Sum
  Add2 : Sum
  Gain : Gain  Gain=0.5
  Gain1 : Gain  Gain=0.5
  Gain2 : Gain  Gain=1/4
  Index Vector : MultiPortSwitch  Inputs=6
  Index Vector1 : MultiPortSwitch  Inputs=6
  Index Vector2 : MultiPortSwitch  Inputs=6
  Scope2 : Scope  NumInputPorts=3
  Tcm1 : Outport
  Tcm2 : Outport  Port=2
  Tcm3 : Outport  Port=3
  wires:
  Index Vector2/1 -> Scope2/3, Tcm3/1
  N/1 -> Index Vector/1, Index Vector1/1, Index Vector2/1
  Add2/1 -> Index Vector/5, Index Vector/6, Index Vector1/3, Index Vector1/7, Index Vector2/2, Index Vector2/4
  Gain1/1 -> Add2/1
  Add1/1 -> Add2/2, Index Vector/2, Index Vector/7, Index Vector1/4, Index Vector1/5, Index Vector2/3, Index Vector2/6
  Gain2/1 -> Index Vector2/5, Index Vector2/7, Add1/2, Index Vector/3, Index Vector/4, Index Vector1/2, Index Vector1/6
  Gain/1 -> Add1/1
  Add/1 -> Gain2/1
  Tpwm/1 -> Add/3
  T2/1 -> Add/2, Gain1/1
  T1/1 -> Add/1, Gain/1
  Index Vector/1 -> Scope2/1, Tcm1/1
  Index Vector1/1 -> Scope2/2, Tcm2/1

== system PMSM_FOC_Tractio/Motor_Control/Motor_Control_Funtion/FOC_Control_100us/FOC/SVPWM/XYZ Caculate ==
  note: X
  note: Y
  note: Z
  Ualfpa : Inport
  Ubelta : Inport  Port=2
  Udc : Inport  Port=3
  Tpwm : Inport  Port=4
  Add1 : Sum  Inputs=-+
  Add2 : Sum  Inputs=--
  Constant : Constant  Value=sqrt(3)  OutDataTypeStr=single
  Divide : Product  Inputs=**/
  Gain : Gain  Gain=sqrt(3)
  Gain1 : Gain  Gain=-0.5
  Gain2 : Gain  Gain=-0.5
  Product : Product
  Product1 : Product
  Product2 : Product
  X : Outport
  Y : Outport  Port=2
  Z : Outport  Port=3
  wires:
  Gain2/1 -> Product1/1
  Add2/1 -> Gain2/1
  Add1/1 -> Gain1/1
  Gain/1 -> Add2/2, Add1/2
  Ualfpa/1 -> Gain/1
  Ubelta/1 -> Add2/1, Add1/1, Product/1
  Gain1/1 -> Product2/2
  Product2/1 -> Z/1
  Divide/1 -> Product1/2, Product2/1, Product/2
  Product1/1 -> Y/1
  Product/1 -> X/1
  Udc/1 -> Divide/3
  Tpwm/1 -> Divide/2
  Constant/1 -> Divide/1

== system PMSM_FOC_Tractio/Motor_Control/Motor_Control_Funtion/FOC_Control_100us/FOC/Set_Idq/Set_Idq ==
  Id_Command : Inport
  Iq_Command : Inport  Port=2
  Action Port : ActionPort  ActionPortLabel=if(u1==2 | u1==1)
  Id : Outport  VectorParamsAs1DForOutWhenUnconnected=off
  Iq : Outport  Port=2  VectorParamsAs1DForOutWhenUnconnected=off
  wires:
  Id_Command/1 -> Id/1
  Iq_Command/1 -> Iq/1

== system PMSM_FOC_Tractio/Motor_Control/Motor_Control_Funtion/FOC_Control_100us/FOC/Set_Idq/Set_Idq1 ==
  Id_Command : Inport
  Iq_Command : Inport  Port=2
  Action Port : ActionPort  ActionPortLabel=else
  Id : Outport  VectorParamsAs1DForOutWhenUnconnected=off
  Iq : Outport  Port=2  VectorParamsAs1DForOutWhenUnconnected=off
  wires:
  Id_Command/1 -> Id/1
  Iq_Command/1 -> Iq/1

== system PMSM_FOC_Tractio/Motor_Control/Motor_Control_Funtion/FOC_Control_100us/FOC/Subsystem1/If Action Subsystem1 ==
  In1 : Inport
  In2 : Inport  Port=2
  Action Port : ActionPort  ActionPortLabel=else
  Out1 : Outport
  Out2 : Outport  Port=2
  wires:
  In1/1 -> Out1/1
  In2/1 -> Out2/1

== system PMSM_FOC_Tractio/Motor_Control/Motor_Control_Funtion/FOC_Control_100us/FOC/Subsystem1/If Action Subsystem2 ==
  In1 : Inport
  In2 : Inport  Port=2
  Action Port : ActionPort  ActionPortLabel=if((u1<3)&(u1>0))
  Out1 : Outport
  Out2 : Outport  Port=2
  wires:
  In1/1 -> Out1/1
  In2/1 -> Out2/1

== system PMSM_FOC_Tractio/Motor_Control/Motor_Control_Funtion/Angle_Speed_100us/SpeedAndAngle/ACC_OMG/BLDC/Control ==
  RPMReq : Inport
  w_sens : Inport  Port=2
  Hall : Inport  Port=3
  BLDC_State : Inport  Port=4
  Commutation : Subsystem
  If1 : If  IfExpression=u1==3  ShowElse=off
  Scope3 : Scope
  Speed_Control : Subsystem
  Sum : Sum  Inputs=|+-
  rad/s->rpm : Gain  Gain=30/pi
  Gate : Outport  VectorParamsAs1DForOutWhenUnconnected=off
  Duty : Outport  Port=2  VectorParamsAs1DForOutWhenUnconnected=off
  wires:
  RPMReq/1 -> Sum/1
  w_sens/1 -> rad/s->rpm/1
  rad/s->rpm/1 -> Sum/2, Scope3/1
  Commutation/1(S) -> Gate/1
  Hall/1 -> Commutation/1(Hall)
  Sum/1 -> Speed_Control/1(Err)
  Speed_Control/1(PI_Out) -> Duty/1
  BLDC_State/1 -> If1/1
  If1/1 -> Speed_Control/Action

== system PMSM_FOC_Tractio/Motor_Control/Motor_Control_Funtion/Angle_Speed_100us/SpeedAndAngle/ACC_OMG/Six_point/Sector_1 ==
  Action Port : ActionPort  ActionPortLabel=case [ 1 ]:
  Add : Sum
  Constant : Constant  Value=Hall_Parameter.Sector_1  OutDataTypeStr=single
  Constant1 : Constant  Value=Hall_Parameter.shift  OutDataTypeStr=single
  Angle_0 : Outport
  wires:
  Constant/1 -> Add/1
  Constant1/1 -> Add/2
  Add/1 -> Angle_0/1

== system PMSM_FOC_Tractio/Motor_Control/Motor_Control_Funtion/Angle_Speed_100us/SpeedAndAngle/ACC_OMG/Six_point/Sector_2 ==
  Action Port : ActionPort  ActionPortLabel=case [ 2 ]:
  Add : Sum
  Constant1 : Constant  Value=Hall_Parameter.shift  OutDataTypeStr=single
  Pi/3 : Constant  Value=Hall_Parameter.Sector_2  OutDataTypeStr=single
  Angle_0 : Outport
  wires:
  Pi/3/1 -> Add/1
  Constant1/1 -> Add/2
  Add/1 -> Angle_0/1

== system PMSM_FOC_Tractio/Motor_Control/Motor_Control_Funtion/Angle_Speed_100us/SpeedAndAngle/ACC_OMG/Six_point/Sector_3 ==
  Action Port : ActionPort  ActionPortLabel=case [ 3 ]:
  Add : Sum
  Constant : Constant  Value=Hall_Parameter.Sector_3  OutDataTypeStr=single
  Constant1 : Constant  Value=Hall_Parameter.shift  OutDataTypeStr=single
  Angle_0 : Outport
  wires:
  Constant/1 -> Add/1
  Add/1 -> Angle_0/1
  Constant1/1 -> Add/2

== system PMSM_FOC_Tractio/Motor_Control/Motor_Control_Funtion/Angle_Speed_100us/SpeedAndAngle/ACC_OMG/Six_point/Sector_4 ==
  Action Port : ActionPort  ActionPortLabel=case [ 4 ]:
  Add : Sum
  Constant : Constant  Value=Hall_Parameter.Sector_4  OutDataTypeStr=single
  Constant1 : Constant  Value=Hall_Parameter.shift  OutDataTypeStr=single
  Angle_0 : Outport
  wires:
  Constant/1 -> Add/1
  Add/1 -> Angle_0/1
  Constant1/1 -> Add/2

== system PMSM_FOC_Tractio/Motor_Control/Motor_Control_Funtion/Angle_Speed_100us/SpeedAndAngle/ACC_OMG/Six_point/Sector_5 ==
  Action Port : ActionPort  ActionPortLabel=case [ 5 ]:
  Add : Sum
  Constant : Constant  Value=Hall_Parameter.Sector_5  OutDataTypeStr=single
  Constant1 : Constant  Value=Hall_Parameter.shift  OutDataTypeStr=single
  Angle_0 : Outport
  wires:
  Constant/1 -> Add/1
  Add/1 -> Angle_0/1
  Constant1/1 -> Add/2

== system PMSM_FOC_Tractio/Motor_Control/Motor_Control_Funtion/Angle_Speed_100us/SpeedAndAngle/ACC_OMG/Six_point/Sector_6 ==
  Action Port : ActionPort  ActionPortLabel=case [ 6 ]:
  Add : Sum
  Constant : Constant  Value=Hall_Parameter.Sector_6  OutDataTypeStr=single
  Constant1 : Constant  Value=Hall_Parameter.shift  OutDataTypeStr=single
  Angle_0 : Outport
  wires:
  Constant/1 -> Add/1
  Add/1 -> Angle_0/1
  Constant1/1 -> Add/2

== system PMSM_FOC_Tractio/Motor_Control/Motor_Control_Funtion/Angle_Speed_100us/SpeedAndAngle/ADC_IRQ/HallAngle_calibration/If Action Subsystem1 ==
  In1 : Inport
  Action Port : ActionPort  ActionPortLabel=else
  Out1 : Outport
  wires:
  In1/1 -> Out1/1

== system PMSM_FOC_Tractio/Motor_Control/Motor_Control_Funtion/Angle_Speed_100us/SpeedAndAngle/ADC_IRQ/HallAngle_calibration/If Action Subsystem2 ==
  In1 : Inport
  Action Port : ActionPort  ActionPortLabel=if(u1 > 6.283185307)
  2pi : Constant  Value=2*pi  OutDataTypeStr=single
  Subtract1 : Sum  Inputs=+-  OutDataTypeStr=single
  Out1 : Outport
  wires:
  In1/1 -> Subtract1/1
  Subtract1/1 -> Out1/1
  2pi/1 -> Subtract1/2

== system PMSM_FOC_Tractio/Motor_Control/Motor_Control_Funtion/Angle_Speed_100us/SpeedAndAngle/ADC_IRQ/HallAngle_calibration/If Action Subsystem3 ==
  In1 : Inport
  Action Port : ActionPort  ActionPortLabel=elseif(u1<0)
  Angle_offset : Constant  Value=2*pi  OutDataTypeStr=single
  Subtract1 : Sum
  Out1 : Outport
  wires:
  In1/1 -> Subtract1/1
  Subtract1/1 -> Out1/1
  Angle_offset/1 -> Subtract1/2

== system PMSM_FOC_Tractio/Motor_Control/Motor_Control_Funtion/Angle_Speed_100us/SpeedAndAngle/Subsystem/Subsystem/Commutation ==
  Bias : Bias  Bias=-1
  Constant : Constant  OutDataTypeStr=double
  Direct Lookup Table (n-D)2 : LookupNDDirect  InputsSelectThisObjectFromTable=Vector  Table=[0 0 0 1 1 0;0 1 1 0 0 0;0 1 0 0 0 1;1 0 0 0 1 0;1 0 1 0 0 0;0 0 0 1 0 1]
  Scope : Scope
  S : Outport  VectorParamsAs1DForOutWhenUnconnected=off
  wires:
  Direct Lookup Table (n-D)2/1 -> S/1
  Constant/1 -> Bias/1
  Bias/1 -> Scope/1, Direct Lookup Table (n-D)2/1

== system PMSM_FOC_Tractio/Motor_Control/Motor_Control_Funtion/Angle_Speed_100us/SpeedAndAngle/Subsystem/Subsystem1/Commutation ==
  Hall : Inport
  Bias : Bias  Bias=-1
  Bit concatenate : Subsystem
  Data Type Conversion : DataTypeConversion
  Direct Lookup Table (n-D)2 : LookupNDDirect  InputsSelectThisObjectFromTable=Vector  Table=[0 0 0 1 1 0;0 1 1 0 0 0;0 1 0 0 0 1;1 0 0 0 1 0;1 0 1 0 0 0;0 0 0 1 0 1]
  Scope : Scope
  S : Outport  VectorParamsAs1DForOutWhenUnconnected=off
  wires:
  Hall/1 -> Bit concatenate/1(u)
  Bit concatenate/1(y) -> Data Type Conversion/1
  Direct Lookup Table (n-D)2/1 -> S/1
  Data Type Conversion/1 -> Bias/1
  Bias/1 -> Scope/1, Direct Lookup Table (n-D)2/1
